simulink model "Sistema5 (1)"  (R2023a)
settings: Solver=VariableStepAuto  StartTime=0.0  StopTime=10  RelTol=1e-3
libraries: slpidlib x2
settings Model: Creator=darkn  LastModifiedBy=User
settings DebuggingCC: AlgebraicLoopMsg=none

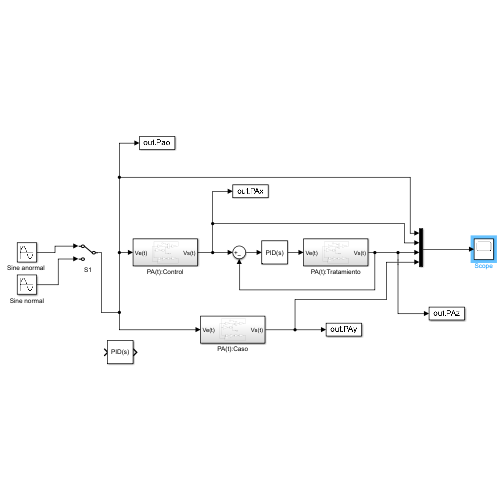
[thumbnail: Simulink's stored preview of the top-level diagram]
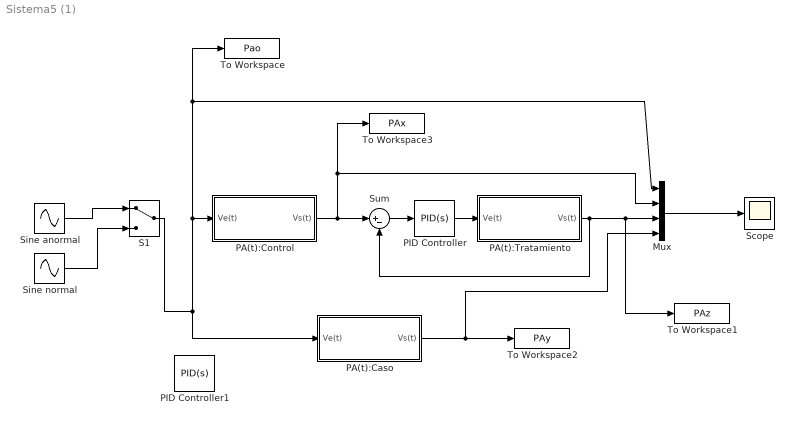
== system Sistema5 (1) ==
  Mux : Mux
  PA(t):Caso : Subsystem
  PA(t):Control : Subsystem
  PA(t):Tratamiento : Subsystem
  PID Controller : slpidlib/PID Controller  Controller=PID  Form=Parallel  TimeDomain=Continuous-time  UseExternalTs=off  SampleTime=-1  IntegratorMethod=Forward Euler  FilterMethod=Forward Euler  ControllerParametersSource=internal  P=130.872808151015  I=3142.46144364491  UseKiTs=off  D=0.108867024129701  N=729.649524900008  UseFilter=on  TunerSelectOption=Transfer Function Based (PID Tuner App)  InitialConditionSource=internal  InitialConditionForIntegrator=0  InitialConditionForFilter=0  DifferentiatorICPrevScaledInput=0  ExternalReset=none  TrackingMode=off  Kt=1  LimitOutput=off  SatLimitsSource=internal  UpperSaturationLimit=inf  LowerSaturationLimit=-inf  LinearizeAsGain=on  AntiWindupMode=none  Kb=1  LimitIntegrator=off  UpperIntegratorSaturationLimit=inf  LowerIntegratorSaturationLimit=-inf  POutMin=[]  POutMax=[]  IOutMin=[]  IOutMax=[]  DOutMin=[]  DOutMax=[]  NOutMin=[]  NOutMax=[]  SumOutMin=[]  SumOutMax=[]  SaturationOutMin=[]  SaturationOutMax=[]  PParamMin=[]  PParamMax=[]  IParamMin=[]  IParamMax=[]  DParamMin=[]  DParamMax=[]  NParamMin=[]  NParamMax=[]  KbParamMin=[]  KbParamMax=[]  KtParamMin=[]  KtParamMax=[]  KbOutMin=[]  KbOutMax=[]  KtOutMin=[]  KtOutMax=[]  IntegratorOutMin=[]  IntegratorOutMax=[]  FilterOutMin=[]  FilterOutMax=[]  SumI1OutMin=[]  SumI1OutMax=[]  SumI2OutMin=[]  SumI2OutMax=[]  SumI3OutMin=[]  SumI3OutMax=[]  SumI4OutMin=[]  SumI4OutMax=[]  SumDOutMin=[]  SumDOutMax=[]  DifferentiatorOutMin=[]  DifferentiatorOutMax=[]  FilterDiffOutCoefMin=[]  FilterDiffOutCoefMax=[]  ReciprocalOutMin=[]  ReciprocalOutMax=[]  SumDenOutMin=[]  SumDenOutMax=[]  SumNumOutMin=[]  SumNumOutMax=[]  DivideOutMin=[]  DivideOutMax=[]  UdiffTsProdOutMin=[]  UdiffTsProdOutMax=[]  NTsProdOutMin=[]  NTsProdOutMax=[]  UintegralTsProdOutMin=[]  UintegralTsProdOutMax=[]  UngainTsProdOutMin=[]  UngainTsProdOutMax=[]  ClampingZeroOutDataTypeStr=Inherit: Inherit via back propagation  ClampingZeroOutMin=[]  ClampingZeroOutMax=[]  FilterDenConstantOutDataTypeStr=Inherit: Inherit via back propagation  FilterDenConstantOutMin=[]  FilterDenConstantOutMax=[]  PCopyOutDataTypeStr=Inherit: Inherit via back propagation  PCopyOutMin=[]  PCopyOutMax=[]  NCopyOutDataTypeStr=Inherit: Inherit via back propagation  NCopyOutMin=[]  NCopyOutMax=[]  IntegratorContinuousStateAttributes=''  IntegratorStateMustResolveToSignalObject=off  IntegratorRTWStateStorageClass=Auto  FilterContinuousStateAttributes=''  FilterStateMustResolveToSignalObject=off  FilterRTWStateStorageClass=Auto  ParallelPVariant=InternalParameters  IdealPVariant=Disabled  IVariant=InternalParameters  DVariant=InternalParameters  IntegratorVariant=Continuous  SatVariant=Disabled  AWVariant=Passthrough  PCopyVariant=Disabled  TRVariant=Disabled  FdbkBlocksVariant=Forward  IdealPFdbkVariant=Disabled  SatFdbkVariant=Disabled  DerivativeFilterVariant=ContFilter  NVariant=InternalParameters  NCopyVariant=Disabled  FilterICVariant=InternalICsFilter  IntegratorICVariant=InternalICs  ExternalResetVariant=Disabled  TRSumVariant=Passthrough  SumFdbkVariant=Disabled  SumVariant=Sum_PID  TsampFilterVariant=InternalTs  TsampNgainVariant=Passthrough  TsampIntegralVariant=Disabled_SignalSpec  ExternalSaturationOutDataTypeStr=Inherit: Same as second input
  PID Controller1 : slpidlib/PID Controller  Controller=PID  Form=Parallel  TimeDomain=Continuous-time  UseExternalTs=off  SampleTime=-1  IntegratorMethod=Forward Euler  FilterMethod=Forward Euler  ControllerParametersSource=internal  P=204.065571889934  I=3634.73764720607  UseKiTs=off  D=1.0092392750428  N=20647.2985734707  UseFilter=on  TunerSelectOption=Transfer Function Based (PID Tuner App)  InitialConditionSource=internal  InitialConditionForIntegrator=0  InitialConditionForFilter=0  DifferentiatorICPrevScaledInput=0  ExternalReset=none  TrackingMode=off  Kt=1  LimitOutput=off  SatLimitsSource=internal  UpperSaturationLimit=inf  LowerSaturationLimit=-inf  LinearizeAsGain=on  AntiWindupMode=none  Kb=1  LimitIntegrator=off  UpperIntegratorSaturationLimit=inf  LowerIntegratorSaturationLimit=-inf  POutMin=[]  POutMax=[]  IOutMin=[]  IOutMax=[]  DOutMin=[]  DOutMax=[]  NOutMin=[]  NOutMax=[]  SumOutMin=[]  SumOutMax=[]  SaturationOutMin=[]  SaturationOutMax=[]  PParamMin=[]  PParamMax=[]  IParamMin=[]  IParamMax=[]  DParamMin=[]  DParamMax=[]  NParamMin=[]  NParamMax=[]  KbParamMin=[]  KbParamMax=[]  KtParamMin=[]  KtParamMax=[]  KbOutMin=[]  KbOutMax=[]  KtOutMin=[]  KtOutMax=[]  IntegratorOutMin=[]  IntegratorOutMax=[]  FilterOutMin=[]  FilterOutMax=[]  SumI1OutMin=[]  SumI1OutMax=[]  SumI2OutMin=[]  SumI2OutMax=[]  SumI3OutMin=[]  SumI3OutMax=[]  SumI4OutMin=[]  SumI4OutMax=[]  SumDOutMin=[]  SumDOutMax=[]  DifferentiatorOutMin=[]  DifferentiatorOutMax=[]  FilterDiffOutCoefMin=[]  FilterDiffOutCoefMax=[]  ReciprocalOutMin=[]  ReciprocalOutMax=[]  SumDenOutMin=[]  SumDenOutMax=[]  SumNumOutMin=[]  SumNumOutMax=[]  DivideOutMin=[]  DivideOutMax=[]  UdiffTsProdOutMin=[]  UdiffTsProdOutMax=[]  NTsProdOutMin=[]  NTsProdOutMax=[]  UintegralTsProdOutMin=[]  UintegralTsProdOutMax=[]  UngainTsProdOutMin=[]  UngainTsProdOutMax=[]  ClampingZeroOutDataTypeStr=Inherit: Inherit via back propagation  ClampingZeroOutMin=[]  ClampingZeroOutMax=[]  FilterDenConstantOutDataTypeStr=Inherit: Inherit via back propagation  FilterDenConstantOutMin=[]  FilterDenConstantOutMax=[]  PCopyOutDataTypeStr=Inherit: Inherit via back propagation  PCopyOutMin=[]  PCopyOutMax=[]  NCopyOutDataTypeStr=Inherit: Inherit via back propagation  NCopyOutMin=[]  NCopyOutMax=[]  IntegratorContinuousStateAttributes=''  IntegratorStateMustResolveToSignalObject=off  IntegratorRTWStateStorageClass=Auto  FilterContinuousStateAttributes=''  FilterStateMustResolveToSignalObject=off  FilterRTWStateStorageClass=Auto  ParallelPVariant=InternalParameters  IdealPVariant=Disabled  IVariant=InternalParameters  DVariant=InternalParameters  IntegratorVariant=Continuous  SatVariant=Disabled  AWVariant=Passthrough  PCopyVariant=Disabled  TRVariant=Disabled  FdbkBlocksVariant=Forward  IdealPFdbkVariant=Disabled  SatFdbkVariant=Disabled  DerivativeFilterVariant=ContFilter  NVariant=InternalParameters  NCopyVariant=Disabled  FilterICVariant=InternalICsFilter  IntegratorICVariant=InternalICs  ExternalResetVariant=Disabled  TRSumVariant=Passthrough  SumFdbkVariant=Disabled  SumVariant=Sum_PID  TsampFilterVariant=InternalTs  TsampNgainVariant=Passthrough  TsampIntegralVariant=Disabled_SignalSpec  ExternalSaturationOutDataTypeStr=Inherit: Same as second input
  S1 : ManualSwitch
  Scope : Scope
  "Sine anormal " : Sin  Amplitude=2.5  Frequency=pi  SampleTime=0
  Sine normal : Sin  Amplitude=2.5  Frequency=pi/2  SampleTime=0
  Sum : Sum  Inputs=|+-
  To Workspace : ToWorkspace  VariableName=Pao  SampleTime=-1
  To Workspace1 : ToWorkspace  VariableName=PAz  SampleTime=-1
  To Workspace2 : ToWorkspace  VariableName=PAy  SampleTime=-1
  To Workspace3 : ToWorkspace  VariableName=PAx  SampleTime=-1
  wires:
  PA(t):Tratamiento/1(Vs(t)) -> Sum/2, To Workspace1/1, Mux/3
  PID Controller/1 -> PA(t):Tratamiento/1(Ve(t))
  Sum/1 -> PID Controller/1
  Mux/1 -> Scope/1
  PA(t):Caso/1(Vs(t)) -> Mux/4, To Workspace2/1
  PA(t):Control/1(Vs(t)) -> To Workspace3/1, Mux/2, Sum/1
  S1/1 -> PA(t):Caso/1(Ve(t)), PA(t):Control/1(Ve(t)), To Workspace/1, Mux/1
  "Sine anormal "/1 -> S1/1
  Sine normal/1 -> S1/2

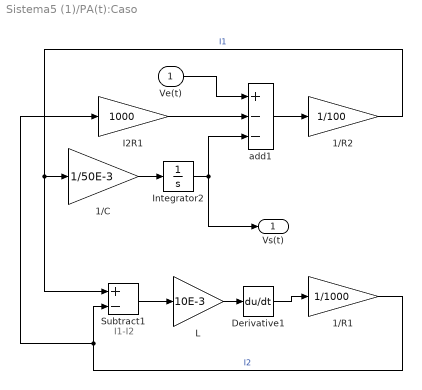
== system Sistema5 (1)/PA(t):Caso ==
  note: I1-I2
  Ve(t) : Inport
  1/C : Gain  Gain=1/50E-3
  1/R1 : Gain  Gain=1/1000
  1/R2 : Gain  Gain=1/100
  Derivative1 : Derivative
  I2R1 : Gain  Gain=1000
  Integrator2 : Integrator
  L : Gain  Gain=10E-3
  Subtract1 : Sum  Inputs=+-
  add1 : Sum  Inputs=+--
  Vs(t) : Outport
  wires:
  add1/1 -> 1/R2/1
  Ve(t)/1 -> add1/1
  I2R1/1 -> add1/2
  Integrator2/1 -> Vs(t)/1, add1/3
  1/C/1 -> Integrator2/1
  1/R2/1 -> Subtract1/1, 1/C/1  "I1"
  1/R1/1 -> Subtract1/2, I2R1/1  "I2"
  Subtract1/1 -> L/1
  L/1 -> Derivative1/1
  Derivative1/1 -> 1/R1/1

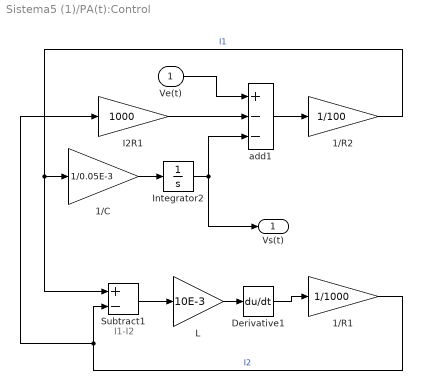
== system Sistema5 (1)/PA(t):Control ==
  note: I1-I2
  Ve(t) : Inport
  1/C : Gain  Gain=1/0.05E-3
  1/R1 : Gain  Gain=1/1000
  1/R2 : Gain  Gain=1/100
  Derivative1 : Derivative
  I2R1 : Gain  Gain=1000
  Integrator2 : Integrator
  L : Gain  Gain=10E-3
  Subtract1 : Sum  Inputs=+-
  add1 : Sum  Inputs=+--
  Vs(t) : Outport
  wires:
  add1/1 -> 1/R2/1
  Ve(t)/1 -> add1/1
  I2R1/1 -> add1/2
  Integrator2/1 -> Vs(t)/1, add1/3
  1/C/1 -> Integrator2/1
  1/R2/1 -> Subtract1/1, 1/C/1  "I1"
  1/R1/1 -> Subtract1/2, I2R1/1  "I2"
  Subtract1/1 -> L/1
  L/1 -> Derivative1/1
  Derivative1/1 -> 1/R1/1

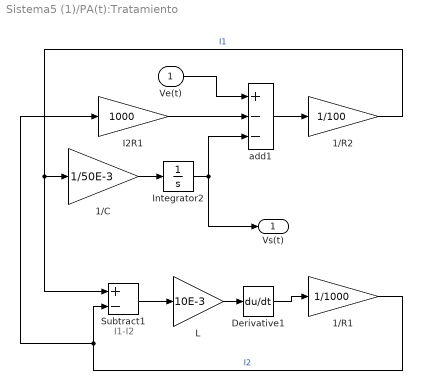
== system Sistema5 (1)/PA(t):Tratamiento ==
  note: I1-I2
  Ve(t) : Inport
  1/C : Gain  Gain=1/50E-3
  1/R1 : Gain  Gain=1/1000
  1/R2 : Gain  Gain=1/100
  Derivative1 : Derivative
  I2R1 : Gain  Gain=1000
  Integrator2 : Integrator
  L : Gain  Gain=10E-3
  Subtract1 : Sum  Inputs=+-
  add1 : Sum  Inputs=+--
  Vs(t) : Outport
  wires:
  add1/1 -> 1/R2/1
  Ve(t)/1 -> add1/1
  I2R1/1 -> add1/2
  Integrator2/1 -> Vs(t)/1, add1/3
  1/C/1 -> Integrator2/1
  1/R2/1 -> Subtract1/1, 1/C/1  "I1"
  1/R1/1 -> Subtract1/2, I2R1/1  "I2"
  Subtract1/1 -> L/1
  L/1 -> Derivative1/1
  Derivative1/1 -> 1/R1/1
